simulink model "bateria (1)"  (R2023a)
settings: Solver=FixedStepAuto  StartTime=0.0  StopTime=3600*3  FixedStep=1  RelTol=1e-3
settings Model: Creator=cesar  LastModifiedBy=cesar

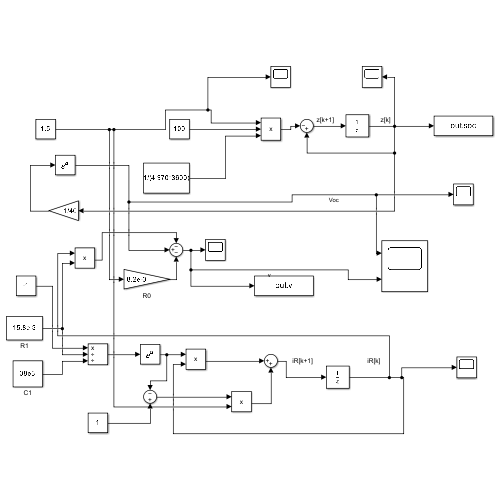
[thumbnail: Simulink's stored preview of the top-level diagram]
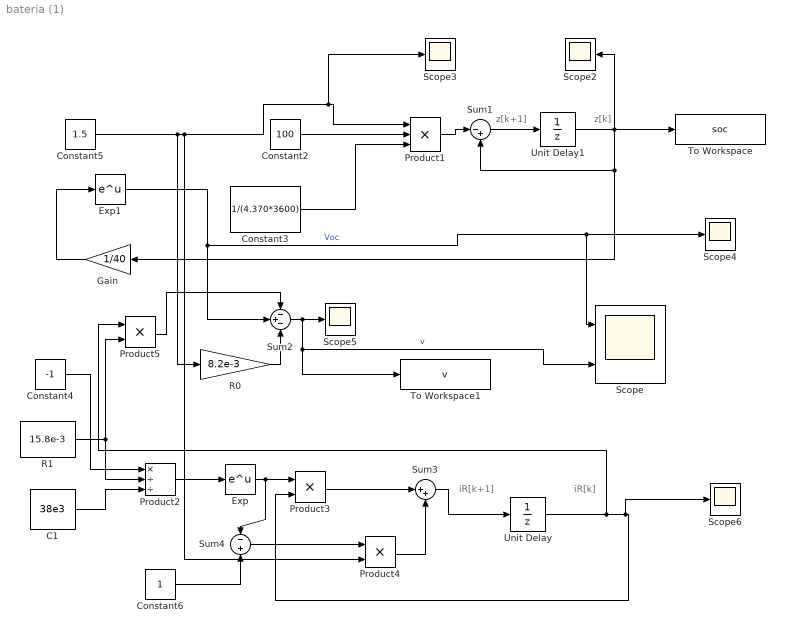
== system bateria (1) ==
  note: iR[k]
  note: iR[k+1]
  note: z[k+1]
  note: z[k]
  C1 : Constant  Value=38e3
  Constant2 : Constant  Value=100
  Constant3 : Constant  Value=1/(4.370*3600)
  Constant4 : Constant  Value=-1
  Constant5 : Constant  Value=1.5
  Constant6 : Constant
  Exp : Math
  Exp1 : Math
  Gain : Gain  Gain=1/40
  Product1 : Product  Inputs=3
  Product2 : Product  Inputs=*//
  Product3 : Product
  Product4 : Product
  Product5 : Product
  R0 : Gain  Gain=8.2e-3
  R1 : Constant  Value=15.8e-3
  Scope : Scope  NumInputPorts=2
  Scope{2..6} (5 alike) : Scope
  Sum1 : Sum  Inputs=|-+
  Sum2 : Sum  Inputs=-+-
  Sum3 : Sum  Inputs=|++
  Sum4 : Sum  Inputs=-+
  To Workspace : ToWorkspace  VariableName=soc  SampleTime=-1
  To Workspace1 : ToWorkspace  VariableName=v  SampleTime=-1
  Unit Delay : UnitDelay  SampleTime=-1  HasFrameUpgradeWarning=on
  Unit Delay1 : UnitDelay  InitialCondition=80  SampleTime=-1  HasFrameUpgradeWarning=on
  wires:
  Product1/1 -> Sum1/1
  Sum1/1 -> Unit Delay1/1
  Constant5/1 -> Product4/2, Scope3/1, Product1/1, R0/1
  Constant3/1 -> Product1/3
  Constant2/1 -> Product1/2
  Gain/1 -> Exp1/1
  Unit Delay1/1 -> To Workspace/1, Scope2/1, Gain/1, Sum1/2
  R0/1 -> Sum2/3
  Sum2/1 -> Scope/2, To Workspace1/1, Scope5/1  "v"
  R1/1 -> Product2/2, Product5/2
  C1/1 -> Product2/3
  Constant4/1 -> Product2/1
  Product2/1 -> Exp/1
  Unit Delay/1 -> Product5/1, Scope6/1, Product3/2
  Exp/1 -> Product3/1, Sum4/1
  Product3/1 -> Sum3/1
  Constant6/1 -> Sum4/2
  Sum4/1 -> Product4/1
  Product4/1 -> Sum3/2
  Sum3/1 -> Unit Delay/1
  Product5/1 -> Sum2/1
  Exp1/1 -> Scope/1, Scope4/1, Sum2/2  "Voc"
